simulink model "simulink_implementation_q30x5B10x5D"  (R2023b)
settings: Solver=VariableStepAuto  StartTime=0.0  StopTime=10.0  RelTol=1e-3
settings Model: Creator=Aman Tripathi  LastModifiedBy=Spedrik Webster

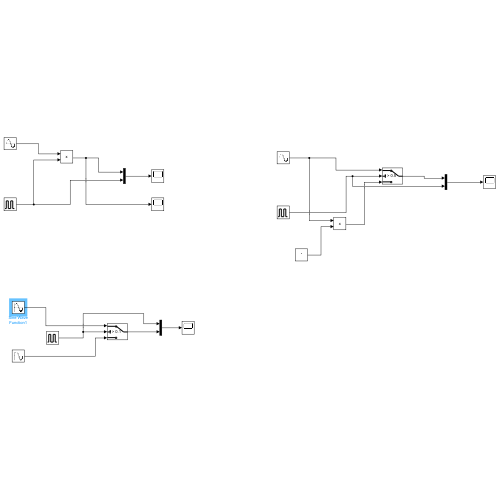
[thumbnail: Simulink's stored preview of the top-level diagram]
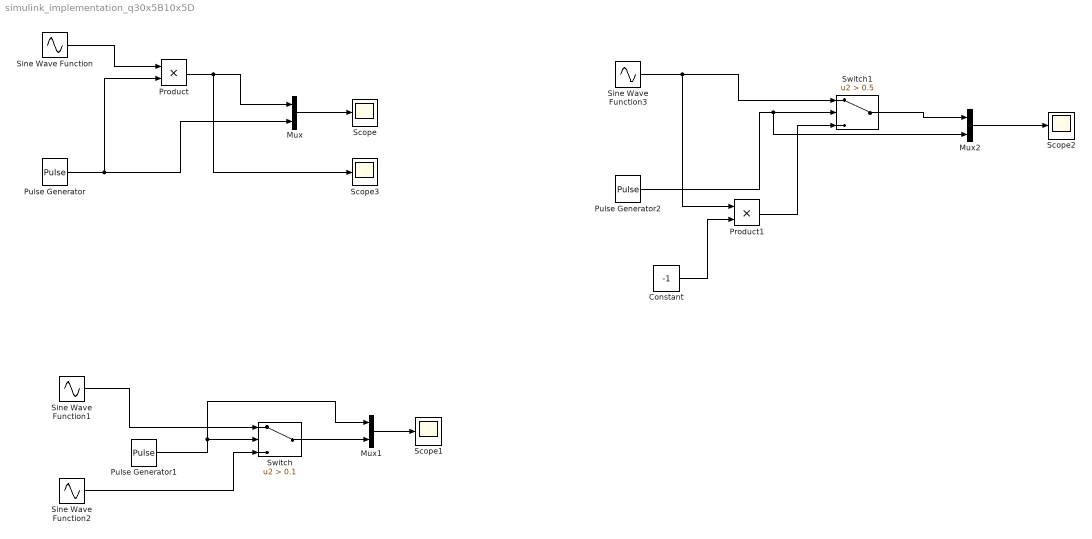
== system simulink_implementation_q30x5B10x5D ==
  Constant : Constant  Value=-1
  Mux : Mux  Inputs=2
  Mux1 : Mux  Inputs=2
  Mux2 : Mux  Inputs=2
  Product : Product
  Product1 : Product
  Pulse Generator : DiscretePulseGenerator  PulseType=Time based  PulseWidth=50
  Pulse Generator1 : DiscretePulseGenerator  PulseType=Time based  PulseWidth=50
  Pulse Generator2 : DiscretePulseGenerator  PulseType=Time based  PulseWidth=50
  Scope{,1..3} (4 alike) : Scope
  Sine Wave Function : Sin  Frequency=50  SampleTime=1/5000
  Sine Wave Function1 : Sin  Frequency=20  SampleTime=1/5000
  Sine Wave Function2 : Sin  Frequency=130  SampleTime=1/5000
  Sine Wave Function3 : Sin  Frequency=10  SampleTime=1/5000
  Switch : Switch  Criteria=u2 > Threshold  Threshold=0.1  SaturateOnIntegerOverflow=off  InputSameDT=off
  Switch1 : Switch  Criteria=u2 > Threshold  Threshold=0.5  SaturateOnIntegerOverflow=off  InputSameDT=off
  wires:
  Sine Wave Function/1 -> Product/1
  Pulse Generator/1 -> Product/2, Mux/2
  Product/1 -> Scope3/1, Mux/1
  Mux/1 -> Scope/1
  Switch/1 -> Mux1/2
  Pulse Generator1/1 -> Switch/2, Mux1/1
  Mux1/1 -> Scope1/1
  Sine Wave Function1/1 -> Switch/1
  Sine Wave Function2/1 -> Switch/3
  Mux2/1 -> Scope2/1
  Constant/1 -> Product1/2
  Sine Wave Function3/1 -> Product1/1, Switch1/1
  Pulse Generator2/1 -> Mux2/2, Switch1/2
  Product1/1 -> Switch1/3
  Switch1/1 -> Mux2/1
